simulink model "partA"  (R2018b)
settings: Solver=VariableStepAuto  StartTime=0.0  StopTime=300  RelTol=1e-3
settings Model: Creator=ms18975  LastModifiedBy=shins

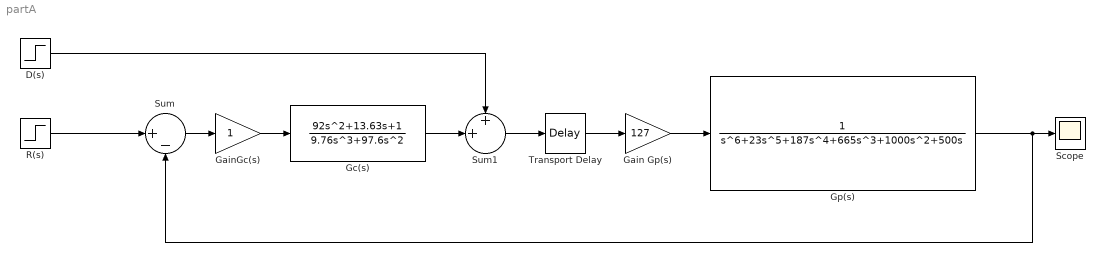
== system partA ==
  D(s) : Step  Time=150  After=0.25  SampleTime=0
  Gain Gp(s) : Gain  Gain=127
  GainGc(s) : Gain
  Gc(s) : TransferFcn  Numerator=[92 13.63 1]  Denominator=[9.76 97.6 0 0]
  Gp(s) : TransferFcn  Denominator=[1 23 187 665 1000 500 0]
  R(s) : Step  Time=0  SampleTime=0
  Scope : Scope
  Sum : Sum  Inputs=|+-
  Sum1 : Sum  Inputs=++|
  Transport Delay : TransportDelay  DelayTime=0.2
  wires:
  R(s)/1 -> Sum/1
  Transport Delay/1 -> Gain Gp(s)/1
  Sum/1 -> GainGc(s)/1
  Gc(s)/1 -> Sum1/2
  Gp(s)/1 -> Sum/2, Scope/1
  Sum1/1 -> Transport Delay/1
  D(s)/1 -> Sum1/1
  Gain Gp(s)/1 -> Gp(s)/1
  GainGc(s)/1 -> Gc(s)/1
